simulink library "StreetLanesLibrary"  (R2021a)
settings: Solver=VariableStepAuto  StartTime=0.0  StopTime=10.0  RelTol=1e-3
undefined symbols (not defined in the file): x0z, xz, yin, yout, yz
libraries: $bdroot x4
settings Model: Creator=phill  LastModifiedBy=phill

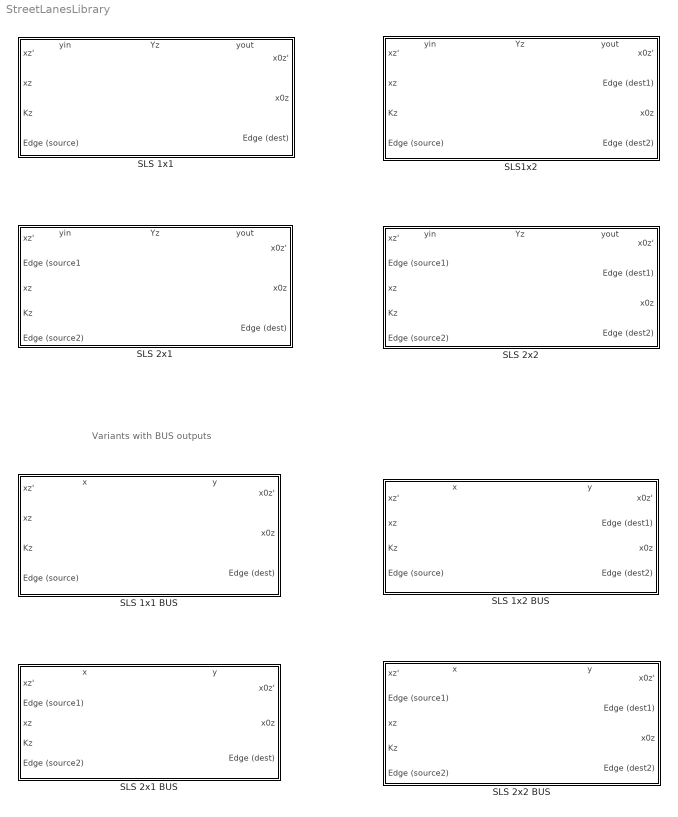
== system StreetLanesLibrary ==
  note: Variants with BUS outputs
  SLS 1x1 : Subsystem  mask{Kz=0, Tz=0}
      mask prompts: Kz "Kz (Capacity - How many cars fit into this cell)"; Tz "Tz (Nominal travel time for vehicles traveling unobstructed through the cell)"
      mask help:
      | This Block models a single Street-Lane capable of holding / transducing cars (or at least "car volume units") as a cell. This 1x1 version It is connected to a single source edge (over which it can receive cars from a preceeding cell) and a single destination edge (over which it can lose cars to the succeeding cell).  It has a capacity (how many volume-units of cars can be present on the segment at a given time) and a nominal travel time (how long cars would need to travel through it unobstructed). The outputs are:
      |
      | x0z  : how many cars (in car volume units) are "at the end of the cell" (and thus visible for the destination-edge  or the following cell).  The value can only rise if more cars flow in (mind the delay Tz!) than flow out - for instance if a traffic light blocks the exit.
      | x0z' : the rate of change for the number of cars "at the end of the cell". Will be positive when more cars arrive than drive out, and negative when more cars leave it.
      | xz    : how many cars are in the cell in total (both the ones who just entered and have not reached the end yet, as well as the ones at the end)
      | xz'   : how many cars are flowing into- (positive sign) or out of (negative) the cell per time
      | yz    : the internal flow - how many cars pass into the "endpart" of a cell. It is delayed by Tz compared to the incoming flow y_incoming, so any cars that enter a cell will only "appear visible" at the end of it after that time Tz.
      | yin : the total flow of cars into the cell
      | yout : the total flow of cars out of the cell
      settings: PortSchema="{\"entries\":[{\"content\":{\"sides\":[{\"content\":{\"connectorIds\":[\"Out6\",\"Out7\",\"Out8\",\"In1\"]},\"type\":\"ConnectorPlacement.EquallySpacedRectSide\",\"uuid\":\"b56112e8-b85b-4d96-b16e-87da935c2eb5\"},{\"content\":{\"connectorIds\":[\"Out1\",\"Out2\",\"In2\"],\"side\":\"RIGHT\"},\"type\":\"ConnectorPlacement.EquallySpacedRectSide\",\"uuid\":\"b630fa9f-2c61-4be9-8eda-7801a9181fe6\"},{\"content\":{\"connectorIds\":[\"Out3\",\"Out4\",\"Out5\"],\"side\":\"TOP\"},\"type\":\"ConnectorPlacement.EquallySpacedRectSide\",\"uuid\":\"9228b8fb-3ac5-45dc-984e-353749c7821d\"}]},\"type\":\"ConnectorPlacement.EquallySpacedConnector\",\"uuid\":\"8a64a7aa-d2ee-4eec-8e15-55afacce95b5\"}],\"packageUris\":[\"http://schema.mathworks.com/mf0/Connector/R2020b\"],\"version\":\"1.0\"}"
      mask Display:
      | image('$imagefile'); % Use "Edit Image" on toolstrip to change.
      | %image('$imagefile');
      | disp('Street Lane Segment 1x1 \n\n');
      | disp(['Kz = ', get_param(gcb,'Kz'), ' | Tz = ', get_param(gcb, 'Tz')])
  SLS 1x1 BUS : Subsystem  mask{Kz=0, Tz=0}
      mask prompts: Kz "Kz (Capacity - How many cars fit into this cell)"; Tz "Tz (Nominal travel time for vehicles traveling unobstructed through the cell)"
      mask help:
      | This Block models a single Street-Lane capable of holding / transducing cars (or at least "car volume units") as a cell. This 1x1 version It is connected to a single source edge (over which it can receive cars from a preceeding cell) and a single destination edge (over which it can lose cars to the succeeding cell).  It has a capacity (how many volume-units of cars can be present on the segment at a given time) and a nominal travel time (how long cars would need to travel through it unobstructed). The outputs are:
      |
      | x0z  : how many cars (in car volume units) are "at the end of the cell" (and thus visible for the destination-edge  or the following cell).  The value can only rise if more cars flow in (mind the delay Tz!) than flow out - for instance if a traffic light blocks the exit.
      | x0z' : the rate of change for the number of cars "at the end of the cell". Will be positive when more cars arrive than drive out, and negative when more cars leave it.
      | xz    : how many cars are in the cell in total (both the ones who just entered and have not reached the end yet, as well as the ones at the end)
      | xz'   : how many cars are flowing into- (positive sign) or out of (negative) the cell per time
      | yz    : the internal flow - how many cars pass into the "endpart" of a cell. It is delayed by Tz compared to the incoming flow y_incoming, so any cars that enter a cell will only "appear visible" at the end of it after that time Tz.
      | yin : the total flow of cars into the cell
      | yout : the total flow of cars out of the cell
      settings: PortSchema="{\"entries\":[{\"content\":{\"sides\":[{\"content\":{\"connectorIds\":[\"Out5\",\"Out6\",\"Out7\",\"In1\"]},\"type\":\"ConnectorPlacement.EquallySpacedRectSide\",\"uuid\":\"fa7777a8-ec1a-439f-ac9e-e0ed45345ec6\"},{\"content\":{\"connectorIds\":[\"Out1\",\"Out2\",\"In2\"],\"side\":\"RIGHT\"},\"type\":\"ConnectorPlacement.EquallySpacedRectSide\",\"uuid\":\"1d8f22c6-fff9-419e-a471-d80b757471c2\"},{\"content\":{\"connectorIds\":[\"Out3\",\"Out4\"],\"side\":\"TOP\"},\"type\":\"ConnectorPlacement.EquallySpacedRectSide\",\"uuid\":\"5603a277-4601-4f1d-99e7-cf6c913c8902\"}]},\"type\":\"ConnectorPlacement.EquallySpacedConnector\",\"uuid\":\"948237b2-05cb-41b3-a7da-b6feef56487f\"}],\"packageUris\":[\"http://schema.mathworks.com/mf0/Connector/R2020b\"],\"version\":\"1.0\"}"
      mask Display:
      | image('$imagefile'); % Use "Edit Image" on toolstrip to change.
      | %image('$imagefile');
      | disp('Street Lane Segment 1x1 \n\n');
      | disp(['Kz = ', get_param(gcb,'Kz'), ' | Tz = ', get_param(gcb, 'Tz')])
  SLS 1x2 BUS : Subsystem  mask{Kz=0, Tz=0}
      mask prompts: Kz "Kz (Capacity - How many cars fit into this cell)"; Tz "Tz (Nominal travel time for vehicles traveling unobstructed through the cell)"
      mask help: 1x2 Version of the 1x1 default cell.
      settings: PortSchema="{\"entries\":[{\"content\":{\"sides\":[{\"content\":{\"connectorIds\":[\"Out5\",\"Out6\",\"Out7\",\"In1\"]},\"type\":\"ConnectorPlacement.EquallySpacedRectSide\",\"uuid\":\"95d0121f-acb2-4e25-97c7-15db8ac80d70\"},{\"content\":{\"connectorIds\":[\"Out1\",\"In2\",\"Out2\",\"In3\"],\"side\":\"RIGHT\"},\"type\":\"ConnectorPlacement.EquallySpacedRectSide\",\"uuid\":\"74008a0d-3aff-4b45-b66c-7df902aff109\"},{\"content\":{\"connectorIds\":[\"Out3\",\"Out4\"],\"side\":\"TOP\"},\"type\":\"ConnectorPlacement.EquallySpacedRectSide\",\"uuid\":\"60b01591-4a61-43c7-92fb-9786f4f21d2e\"}]},\"type\":\"ConnectorPlacement.EquallySpacedConnector\",\"uuid\":\"7f6ca8c0-19be-43e0-a232-af4f67956fb4\"}],\"packageUris\":[\"http://schema.mathworks.com/mf0/Connector/R2020b\"],\"version\":\"1.0\"}"
      mask Display:
      | image('$imagefile'); % Use "Edit Image" on toolstrip to change.
      | %image('$imagefile');
      | disp('Street Lane Segment 1x2 \n\n');
      | disp(['Kz = ', get_param(gcb,'Kz'), ' | Tz = ', get_param(gcb, 'Tz')])
  SLS 2x1 : Subsystem  mask{Kz=0, Tz=0}
      mask prompts: Kz "Kz (Capacity - How many cars fit into this cell)"; Tz "Tz (Nominal travel time for vehicles traveling unobstructed through the cell)"
      mask help: The 2x1 version of the basic 1x1 cell
      settings: PortSchema="{\"entries\":[{\"content\":{\"sides\":[{\"content\":{\"connectorIds\":[\"Out6\",\"In1\",\"Out7\",\"Out8\",\"In2\"]},\"type\":\"ConnectorPlacement.EquallySpacedRectSide\",\"uuid\":\"c6485919-43c0-4a3b-9a67-3a50a1748552\"},{\"content\":{\"connectorIds\":[\"Out1\",\"Out2\",\"In3\"],\"side\":\"RIGHT\"},\"type\":\"ConnectorPlacement.EquallySpacedRectSide\",\"uuid\":\"e12fc750-a76b-4a52-a085-56205ebef983\"},{\"content\":{\"connectorIds\":[\"Out3\",\"Out4\",\"Out5\"],\"side\":\"TOP\"},\"type\":\"ConnectorPlacement.EquallySpacedRectSide\",\"uuid\":\"04ec9430-4292-4c0e-9b60-ad78ee5b6ee3\"}]},\"type\":\"ConnectorPlacement.EquallySpacedConnector\",\"uuid\":\"8d657383-4de4-4f3e-906b-2968264a5f3c\"}],\"packageUris\":[\"http://schema.mathworks.com/mf0/Connector/R2020b\"],\"version\":\"1.0\"}"
      mask Display:
      | image('$imagefile'); % Use "Edit Image" on toolstrip to change.
      | %image('$imagefile');
      | disp('Street Lane Segment 2x1 \n\n');
      | disp(['Kz = ', get_param(gcb,'Kz'), ' | Tz = ', get_param(gcb, 'Tz')])
  SLS 2x1 BUS : Subsystem  mask{Kz=0, Tz=0}
      mask prompts: Kz "Kz (Capacity - How many cars fit into this cell)"; Tz "Tz (Nominal travel time for vehicles traveling unobstructed through the cell)"
      mask help: The 2x1 version of the basic 1x1 cell
      settings: PortSchema="{\"entries\":[{\"content\":{\"sides\":[{\"content\":{\"connectorIds\":[\"Out5\",\"In1\",\"Out6\",\"Out7\",\"In2\"]},\"type\":\"ConnectorPlacement.EquallySpacedRectSide\",\"uuid\":\"95d0121f-acb2-4e25-97c7-15db8ac80d70\"},{\"content\":{\"connectorIds\":[\"Out1\",\"Out2\",\"In3\"],\"side\":\"RIGHT\"},\"type\":\"ConnectorPlacement.EquallySpacedRectSide\",\"uuid\":\"74008a0d-3aff-4b45-b66c-7df902aff109\"},{\"content\":{\"connectorIds\":[\"Out3\",\"Out4\"],\"side\":\"TOP\"},\"type\":\"ConnectorPlacement.EquallySpacedRectSide\",\"uuid\":\"60b01591-4a61-43c7-92fb-9786f4f21d2e\"}]},\"type\":\"ConnectorPlacement.EquallySpacedConnector\",\"uuid\":\"7f6ca8c0-19be-43e0-a232-af4f67956fb4\"}],\"packageUris\":[\"http://schema.mathworks.com/mf0/Connector/R2020b\"],\"version\":\"1.0\"}"
      mask Display:
      | image('$imagefile'); % Use "Edit Image" on toolstrip to change.
      | disp('Street Lane Segment 2x1 \n\n');
      | disp(['Kz = ', get_param(gcb,'Kz'), ' | Tz = ', get_param(gcb, 'Tz')])
  SLS 2x2 : Subsystem  mask{Kz=0, Tz=0}
      mask prompts: Kz "Kz (Capacity - How many cars fit into this cell)"; Tz "Tz (Nominal travel time for vehicles traveling unobstructed through the cell)"
      settings: PortSchema="{\"entries\":[{\"content\":{\"sides\":[{\"content\":{\"connectorIds\":[\"Out6\",\"In1\",\"Out7\",\"Out8\",\"In2\"]},\"type\":\"ConnectorPlacement.EquallySpacedRectSide\",\"uuid\":\"25df2790-c866-41ff-9dfe-266b31cf62ba\"},{\"content\":{\"connectorIds\":[\"Out1\",\"In3\",\"Out2\",\"In4\"],\"side\":\"RIGHT\"},\"type\":\"ConnectorPlacement.EquallySpacedRectSide\",\"uuid\":\"25d72334-2b21-4272-a907-00400a727cc8\"},{\"content\":{\"connectorIds\":[\"Out3\",\"Out4\",\"Out5\"],\"side\":\"TOP\"},\"type\":\"ConnectorPlacement.EquallySpacedRectSide\",\"uuid\":\"016a1f1d-ac45-4b29-877f-ff17231147ed\"}]},\"type\":\"ConnectorPlacement.EquallySpacedConnector\",\"uuid\":\"d9a39936-9630-4e37-953d-f1129270bc17\"}],\"packageUris\":[\"http://schema.mathworks.com/mf0/Connector/R2020b\"],\"version\":\"1.0\"}"
      mask Display:
      | image('$imagefile'); % Use "Edit Image" on toolstrip to change.
      | %image('$imagefile');
      | disp('Street Lane Segment 2x2 \n\n');
      | disp(['Kz = ', get_param(gcb,'Kz'), ' | Tz = ', get_param(gcb, 'Tz')])
  SLS 2x2 BUS : Subsystem  mask{Kz=0, Tz=0}
      mask prompts: Kz "Kz (Capacity - How many cars fit into this cell)"; Tz "Tz (Nominal travel time for vehicles traveling unobstructed through the cell)"
      mask help: The 2x2 extension to the basic cell.
      settings: PortSchema="{\"entries\":[{\"content\":{\"sides\":[{\"content\":{\"connectorIds\":[\"Out5\",\"In1\",\"Out6\",\"Out7\",\"In2\"]},\"type\":\"ConnectorPlacement.EquallySpacedRectSide\",\"uuid\":\"0d72bc7f-f65e-4e07-ad8f-8c66e41d5ec5\"},{\"content\":{\"connectorIds\":[\"Out1\",\"In3\",\"Out2\",\"In4\"],\"side\":\"RIGHT\"},\"type\":\"ConnectorPlacement.EquallySpacedRectSide\",\"uuid\":\"af462cdf-0fa0-460f-8030-ea00e806c044\"},{\"content\":{\"connectorIds\":[\"Out3\",\"Out4\"],\"side\":\"TOP\"},\"type\":\"ConnectorPlacement.EquallySpacedRectSide\",\"uuid\":\"2548bddb-6962-4693-916e-1100869f2661\"}]},\"type\":\"ConnectorPlacement.EquallySpacedConnector\",\"uuid\":\"37811e3d-8b76-462d-b137-4aea1b95b5f4\"}],\"packageUris\":[\"http://schema.mathworks.com/mf0/Connector/R2020b\"],\"version\":\"1.0\"}"
      mask Display:
      | image('$imagefile'); % Use "Edit Image" on toolstrip to change.
      | disp('Street Lane Segment 2x2 \n\n');
      | disp(['Kz = ', get_param(gcb,'Kz'), ' | Tz = ', get_param(gcb, 'Tz')])
  SLS1x2 : Subsystem  mask{Kz=0, Tz=0}
      mask prompts: Kz "Kz (Capacity - How many cars fit into this cell)"; Tz "Tz (Nominal travel time for vehicles traveling unobstructed through the cell)"
      mask help: 1x2 Version of the 1x1 default cell.
      settings: PortSchema="{\"entries\":[{\"content\":{\"sides\":[{\"content\":{\"connectorIds\":[\"Out6\",\"Out7\",\"Out8\",\"In1\"]},\"type\":\"ConnectorPlacement.EquallySpacedRectSide\",\"uuid\":\"c6485919-43c0-4a3b-9a67-3a50a1748552\"},{\"content\":{\"connectorIds\":[\"Out1\",\"In2\",\"Out2\",\"In3\"],\"side\":\"RIGHT\"},\"type\":\"ConnectorPlacement.EquallySpacedRectSide\",\"uuid\":\"e12fc750-a76b-4a52-a085-56205ebef983\"},{\"content\":{\"connectorIds\":[\"Out3\",\"Out4\",\"Out5\"],\"side\":\"TOP\"},\"type\":\"ConnectorPlacement.EquallySpacedRectSide\",\"uuid\":\"04ec9430-4292-4c0e-9b60-ad78ee5b6ee3\"}]},\"type\":\"ConnectorPlacement.EquallySpacedConnector\",\"uuid\":\"8d657383-4de4-4f3e-906b-2968264a5f3c\"}],\"packageUris\":[\"http://schema.mathworks.com/mf0/Connector/R2020b\"],\"version\":\"1.0\"}"
      mask Display:
      | image('$imagefile'); % Use "Edit Image" on toolstrip to change.
      | %image('$imagefile');
      | disp('Street Lane Segment 1x2 \n\n');
      | disp(['Kz = ', get_param(gcb,'Kz'), ' | Tz = ', get_param(gcb, 'Tz')])

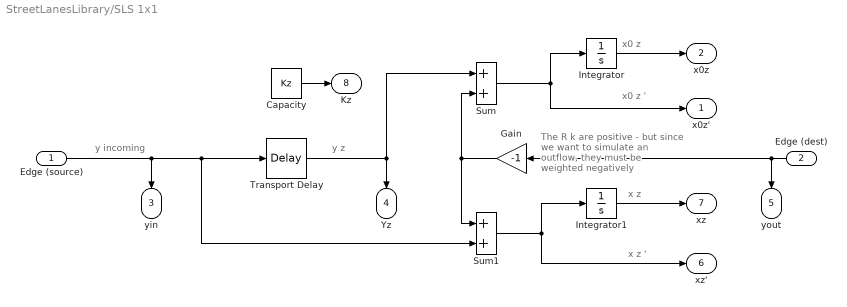
== system StreetLanesLibrary/SLS 1x1 ==
  note: The R k are positive - but since we
      | want to simulate an outflow, they
      | must be weighted negatively
  note: y z
  note: x0 z '
  note: x0 z
  note: x z
  note: x z '
  note: y incoming
  Edge (source) : Inport
  Edge (dest) : Inport  Port=2
  Capacity : Constant  Value=Kz
  Gain : Gain  Gain=-1
  Integrator : Integrator
  Integrator1 : Integrator
  Sum : Sum
  Sum1 : Sum
  Transport Delay : TransportDelay  DelayTime=Tz
  x0z' : Outport
  x0z : Outport  Port=2
  yin : Outport  Port=3
  Yz : Outport  Port=4
  yout : Outport  Port=5
  xz' : Outport  Port=6
  xz : Outport  Port=7
  Kz : Outport  Port=8
  wires:
  Capacity/1 -> Kz/1
  Sum/1 -> Integrator/1, x0z'/1
  Gain/1 -> Sum/2, Sum1/1
  Integrator1/1 -> xz/1
  Edge (source)/1 -> Transport Delay/1, Sum1/2, yin/1
  Edge (dest)/1 -> yout/1, Gain/1
  Transport Delay/1 -> Sum/1, Yz/1
  Integrator/1 -> x0z/1
  Sum1/1 -> Integrator1/1, xz'/1

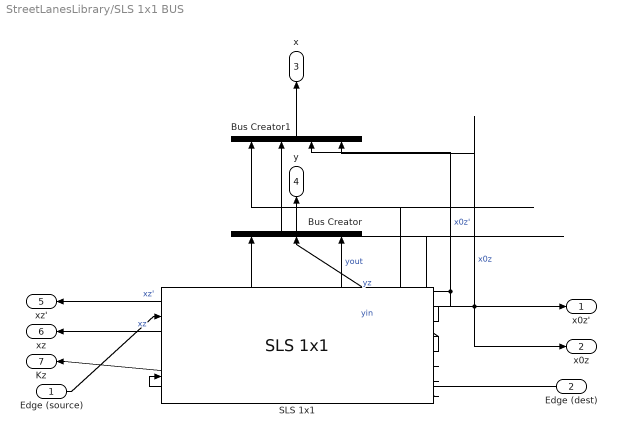
== system StreetLanesLibrary/SLS 1x1 BUS ==
  Edge (source) : Inport
  Edge (dest) : Inport  Port=2
  Bus Creator : BusCreator  Inputs=yin,yz,yout
  Bus Creator1 : BusCreator  Inputs=xz,xz',x0z',x0z
  SLS 1x1 : $bdroot/SLS 1x1  Kz=0  Tz=0
  x0z' : Outport
  x0z : Outport  Port=2
  x : Outport  Port=3
  y : Outport  Port=4
  xz' : Outport  Port=5
  xz : Outport  Port=6
  Kz : Outport  Port=7
  wires:
  Edge (dest)/1 -> SLS 1x1/2
  Edge (source)/1 -> SLS 1x1/1
  SLS 1x1/4 -> Bus Creator/2  "yz"
  Bus Creator1/1 -> x/1
  SLS 1x1/3 -> Bus Creator/1  "yin"
  Bus Creator/1 -> y/1
  SLS 1x1/6 -> Bus Creator1/2, xz'/1  "xz'"
  SLS 1x1/7 -> Bus Creator1/1, xz/1  "xz"
  SLS 1x1/2 -> Bus Creator1/4, x0z/1  "x0z"
  SLS 1x1/1 -> Bus Creator1/3, x0z'/1  "x0z'"
  SLS 1x1/5 -> Bus Creator/3  "yout"
  SLS 1x1/8 -> Kz/1

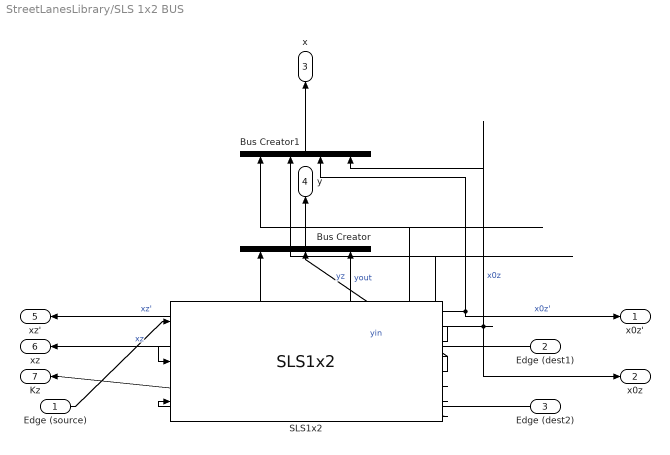
== system StreetLanesLibrary/SLS 1x2 BUS ==
  Edge (source) : Inport
  Edge (dest1) : Inport  Port=2
  Edge (dest2) : Inport  Port=3
  Bus Creator : BusCreator  Inputs=yin,yz,yout
  Bus Creator1 : BusCreator  Inputs=xz,xz',x0z',x0z
  SLS1x2 : $bdroot/SLS1x2  Kz=0  Tz=0
  x0z' : Outport
  x0z : Outport  Port=2
  x : Outport  Port=3
  y : Outport  Port=4
  xz' : Outport  Port=5
  xz : Outport  Port=6
  Kz : Outport  Port=7
  wires:
  Edge (dest2)/1 -> SLS1x2/3
  SLS1x2/8 -> Kz/1
  SLS1x2/1 -> Bus Creator1/3, x0z'/1  "x0z'"
  Edge (dest1)/1 -> SLS1x2/2
  Bus Creator/1 -> y/1
  SLS1x2/7 -> Bus Creator1/1, xz/1  "xz"
  SLS1x2/4 -> Bus Creator/2  "yz"
  SLS1x2/5 -> Bus Creator/3  "yout"
  SLS1x2/3 -> Bus Creator/1  "yin"
  Edge (source)/1 -> SLS1x2/1
  Bus Creator1/1 -> x/1
  SLS1x2/2 -> Bus Creator1/4, x0z/1  "x0z"
  SLS1x2/6 -> Bus Creator1/2, xz'/1  "xz'"

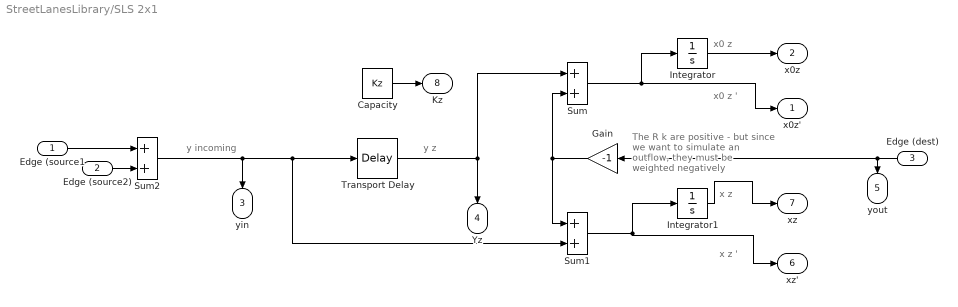
== system StreetLanesLibrary/SLS 2x1 ==
  note: x0 z '
  note: x z '
  note: The R k are positive - but since we
      | want to simulate an outflow, they
      | must be weighted negatively
  note: x z
  note: y incoming
  note: x0 z
  note: y z
  Edge (source1 : Inport
  Edge (source2) : Inport  Port=2
  Edge (dest) : Inport  Port=3
  Capacity : Constant  Value=Kz
  Gain : Gain  Gain=-1
  Integrator : Integrator
  Integrator1 : Integrator
  Sum : Sum
  Sum1 : Sum
  Sum2 : Sum
  Transport Delay : TransportDelay  DelayTime=Tz
  x0z' : Outport
  x0z : Outport  Port=2
  yin : Outport  Port=3
  Yz : Outport  Port=4
  yout : Outport  Port=5
  xz' : Outport  Port=6
  xz : Outport  Port=7
  Kz : Outport  Port=8
  wires:
  Edge (source1/1 -> Sum2/1
  Sum1/1 -> Integrator1/1, xz'/1
  Edge (source2)/1 -> Sum2/2
  Integrator1/1 -> xz/1
  Sum2/1 -> Transport Delay/1, Sum1/2, yin/1
  Edge (dest)/1 -> Gain/1, yout/1
  Gain/1 -> Sum/2, Sum1/1
  Capacity/1 -> Kz/1
  Integrator/1 -> x0z/1
  Sum/1 -> Integrator/1, x0z'/1
  Transport Delay/1 -> Sum/1, Yz/1

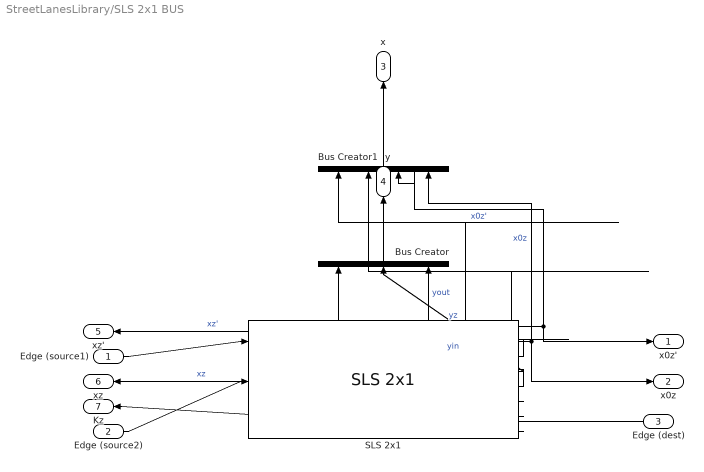
== system StreetLanesLibrary/SLS 2x1 BUS ==
  Edge (source1) : Inport
  Edge (source2) : Inport  Port=2
  Edge (dest) : Inport  Port=3
  Bus Creator : BusCreator  Inputs=yin,yz,yout
  Bus Creator1 : BusCreator  Inputs=xz,xz',x0z',x0z
  SLS 2x1 : $bdroot/SLS 2x1  Kz=0  Tz=0
  x0z' : Outport
  x0z : Outport  Port=2
  x : Outport  Port=3
  y : Outport  Port=4
  xz' : Outport  Port=5
  xz : Outport  Port=6
  Kz : Outport  Port=7
  wires:
  Edge (dest)/1 -> SLS 2x1/3
  Edge (source2)/1 -> SLS 2x1/2
  SLS 2x1/4 -> Bus Creator/2  "yz"
  SLS 2x1/8 -> Kz/1
  SLS 2x1/6 -> Bus Creator1/2, xz'/1  "xz'"
  SLS 2x1/5 -> Bus Creator/3  "yout"
  Bus Creator1/1 -> x/1
  Edge (source1)/1 -> SLS 2x1/1
  Bus Creator/1 -> y/1
  SLS 2x1/1 -> Bus Creator1/3, x0z'/1  "x0z'"
  SLS 2x1/7 -> Bus Creator1/1, xz/1  "xz"
  SLS 2x1/2 -> Bus Creator1/4, x0z/1  "x0z"
  SLS 2x1/3 -> Bus Creator/1  "yin"

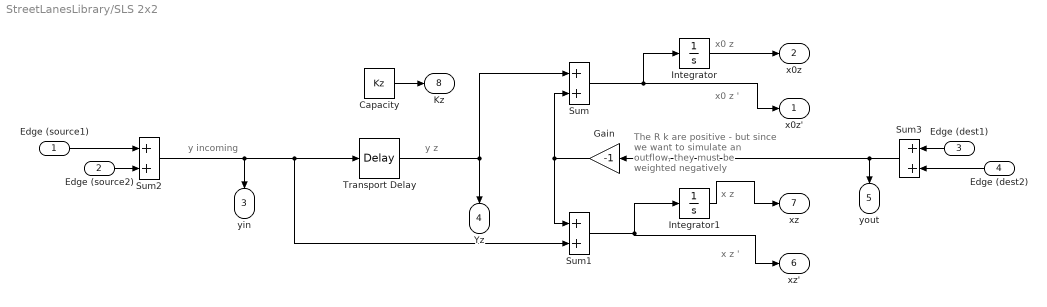
== system StreetLanesLibrary/SLS 2x2 ==
  note: y z
  note: The R k are positive - but since we
      | want to simulate an outflow, they
      | must be weighted negatively
  note: y incoming
  note: x0 z '
  note: x z '
  note: x0 z
  note: x z
  Edge (source1) : Inport
  Edge (source2) : Inport  Port=2
  Edge (dest1) : Inport  Port=3
  Edge (dest2) : Inport  Port=4
  Capacity : Constant  Value=Kz
  Gain : Gain  Gain=-1
  Integrator : Integrator
  Integrator1 : Integrator
  Sum{,1..3} (4 alike) : Sum
  Transport Delay : TransportDelay  DelayTime=Tz
  x0z' : Outport
  x0z : Outport  Port=2
  yin : Outport  Port=3
  Yz : Outport  Port=4
  yout : Outport  Port=5
  xz' : Outport  Port=6
  xz : Outport  Port=7
  Kz : Outport  Port=8
  wires:
  Integrator1/1 -> xz/1
  Edge (dest1)/1 -> Sum3/1
  Gain/1 -> Sum/2, Sum1/1
  Sum/1 -> Integrator/1, x0z'/1
  Edge (dest2)/1 -> Sum3/2
  Sum3/1 -> Gain/1, yout/1
  Sum2/1 -> Transport Delay/1, Sum1/2, yin/1
  Capacity/1 -> Kz/1
  Edge (source1)/1 -> Sum2/1
  Edge (source2)/1 -> Sum2/2
  Sum1/1 -> Integrator1/1, xz'/1
  Transport Delay/1 -> Sum/1, Yz/1
  Integrator/1 -> x0z/1

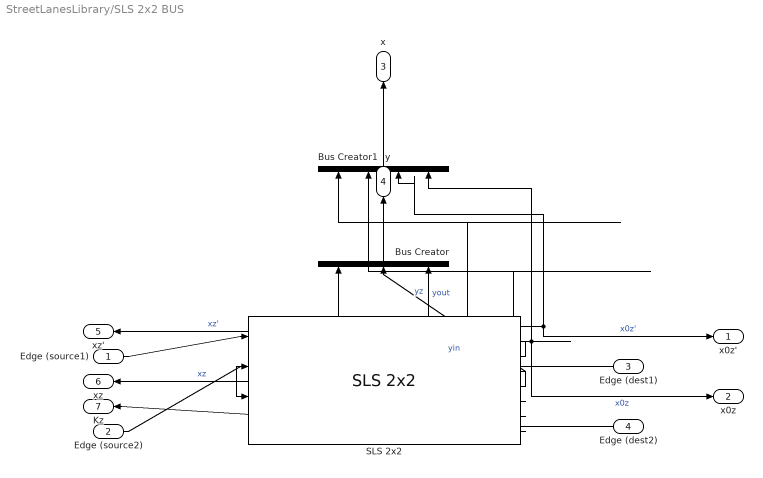
== system StreetLanesLibrary/SLS 2x2 BUS ==
  Edge (source1) : Inport
  Edge (source2) : Inport  Port=2
  Edge (dest1) : Inport  Port=3
  Edge (dest2) : Inport  Port=4
  Bus Creator : BusCreator  Inputs=yin,yz,yout
  Bus Creator1 : BusCreator  Inputs=xz,xz',x0z',x0z
  SLS 2x2 : $bdroot/SLS 2x2  Kz=0  Tz=0
  x0z' : Outport
  x0z : Outport  Port=2
  x : Outport  Port=3
  y : Outport  Port=4
  xz' : Outport  Port=5
  xz : Outport  Port=6
  Kz : Outport  Port=7
  wires:
  Edge (source2)/1 -> SLS 2x2/2
  Edge (dest2)/1 -> SLS 2x2/4
  Edge (dest1)/1 -> SLS 2x2/3
  Edge (source1)/1 -> SLS 2x2/1
  SLS 2x2/3 -> Bus Creator/1  "yin"
  SLS 2x2/4 -> Bus Creator/2  "yz"
  SLS 2x2/5 -> Bus Creator/3  "yout"
  SLS 2x2/2 -> Bus Creator1/4, x0z/1  "x0z"
  SLS 2x2/7 -> Bus Creator1/1, xz/1  "xz"
  SLS 2x2/1 -> Bus Creator1/3, x0z'/1  "x0z'"
  Bus Creator1/1 -> x/1
  SLS 2x2/6 -> Bus Creator1/2, xz'/1  "xz'"
  SLS 2x2/8 -> Kz/1
  Bus Creator/1 -> y/1

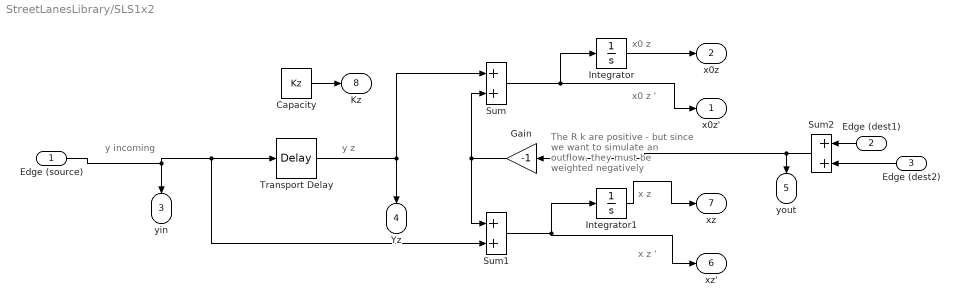
== system StreetLanesLibrary/SLS1x2 ==
  note: x z '
  note: x0 z
  note: x z
  note: y z
  note: y incoming
  note: x0 z '
  note: The R k are positive - but since we
      | want to simulate an outflow, they
      | must be weighted negatively
  Edge (source) : Inport
  Edge (dest1) : Inport  Port=2
  Edge (dest2) : Inport  Port=3
  Capacity : Constant  Value=Kz
  Gain : Gain  Gain=-1
  Integrator : Integrator
  Integrator1 : Integrator
  Sum : Sum
  Sum1 : Sum
  Sum2 : Sum
  Transport Delay : TransportDelay  DelayTime=Tz
  x0z' : Outport
  x0z : Outport  Port=2
  yin : Outport  Port=3
  Yz : Outport  Port=4
  yout : Outport  Port=5
  xz' : Outport  Port=6
  xz : Outport  Port=7
  Kz : Outport  Port=8
  wires:
  Gain/1 -> Sum/2, Sum1/1
  Edge (dest2)/1 -> Sum2/2
  Sum/1 -> Integrator/1, x0z'/1
  Edge (dest1)/1 -> Sum2/1
  Integrator1/1 -> xz/1
  Sum2/1 -> yout/1, Gain/1
  Capacity/1 -> Kz/1
  Transport Delay/1 -> Sum/1, Yz/1
  Integrator/1 -> x0z/1
  Sum1/1 -> Integrator1/1, xz'/1
  Edge (source)/1 -> Transport Delay/1, Sum1/2, yin/1
